simulink model "Ex4_3d"  (R2016b)
settings: Solver=VariableStepAuto  StartTime=0.0  StopTime=50  RelTol=1e-3
values from neighbouring files (symbols this model uses):
  J1 = 1.2    [ex4_3_init.m]
  J2 = 10000    [ex4_3_init.m]
  Ke = 220/50/pi    (= 1.40056349921)    [ex4_3_init.m]
  La = 0.002    [ex4_3_init.m]    (also in ex4_5_init.m = 0.235783633842)
  Ra = 0.05    [ex4_3_init.m]    (also in ex4_5_init.m = 0.1442)
  Re = 2.15    [ex4_3_init.m]
undefined symbols (not defined in the file or in its folder): sigbuilder_block
settings Model: Creator=Niels  LastModifiedBy=Niels

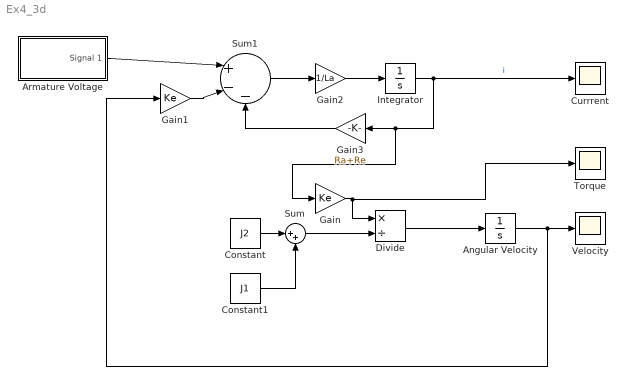
== system Ex4_3d ==
  Angular Velocity : Integrator
  Armature Voltage : Subsystem  Tag=STV Subsys  LoadFcn=sigbuilder_block('load');  StartFcn=sigbuilder_block('start');  StopFcn=sigbuilder_block('stop');  ClipboardFcn=sigbuilder_block('clipboard');  mask(Sigbuilder block){tuvar=[0:10]}
      mask help: Simulink:masks:SigbuilderBlock_MD
      mask init:
      | if ~strcmp(get_param(bdroot(gcbh),'SimulationStatus'),'stopped') tuvar = sigbuilder_block('maskInit'); end
      settings: CopyFcn=sigbuilder_block('copy');  DeleteFcn=sigbuilder_block('delete');  ModelCloseFcn=sigbuilder_block('modelClose');  PreSaveFcn=sigbuilder_block('preSave');  PauseFcn=sigbuilder_block('pause');  ContinueFcn=sigbuilder_block('continue');  NameChangeFcn=sigbuilder_block('namechange');  OpenFcn=sigbuilder_block('open',[437.6 199.2 550.4 400 ]);  CloseFcn=sigbuilder_block('close');
      mask Display: plot(0, 0, 100, 100,[2, 2, 32, 32, 2], [68, 8, 8, 68, 68],[32, 2], [38, 38], [32, 19, 2],[53, 60, 44], [32, 17, 17, 2],[16, 16, 31, 31]);txt = getActiveGroup(gcbh);text(2, 100, txt,'verticalAlignment', 'top');
  Constant : Constant  Value=J2
  Constant1 : Constant  Value=J1
  Currrent : Scope
  Divide : Product  Inputs=*/
  Gain : Gain  Gain=Ke
  Gain1 : Gain  Gain=Ke
  Gain2 : Gain  Gain=1/La
  Gain3 : Gain  Gain=Ra+Re
  Integrator : Integrator
  Sum : Sum  Inputs=|++
  Sum1 : Sum  Inputs=|+--
  Torque : Scope
  "Velocity " : Scope
  wires:
  Constant/1 -> Sum/1
  Constant1/1 -> Sum/2
  Sum/1 -> Divide/2
  Armature Voltage/1(Signal 1) -> Sum1/1
  Gain1/1 -> Sum1/2
  Angular Velocity/1 -> "Velocity "/1, Gain1/1
  Sum1/1 -> Gain2/1
  Gain2/1 -> Integrator/1
  Integrator/1 -> Gain/1, Gain3/1, Currrent/1  "i"
  Gain3/1 -> Sum1/3
  Divide/1 -> Angular Velocity/1
  Gain/1 -> Torque/1, Divide/1

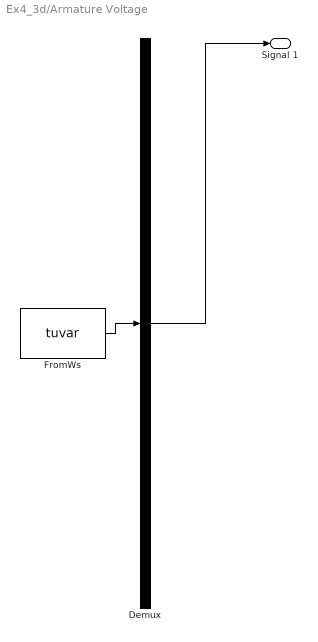
== system Ex4_3d/Armature Voltage ==
  Demux : Demux  Tag=STV Demux  Outputs=1
  FromWs : FromWorkspace  Tag=STV FromWs  VariableName=tuvar  SampleTime=0
      SigBuilderData=|
      | common.afterFinalStr = 'Extrapolate'
      | common.sampleTime = 0
      | dataSet.timeRange = [0 0.5]
      | dataSet.name = 'Group 1'
      | sbobj.Groups.Name = 'Group 1'
      | sbobj.Groups.Signals.Name = 'Signal 1'
      | sbobj.Groups.Signals.XData = [0 0.5]
      | sbobj.Groups.Signals.YData = [220 220]
      | sbobj.Groups.TimeRange = [0 0.5]
  Signal 1 : Outport  Tag=STV Outport
  wires:
  Demux/1 -> Signal 1/1
  FromWs/1 -> Demux/1
